simulink model "lin_mpc_qpoases_inline"  (Simulink 7.8)
settings: Solver=ode45  StartTime=0.0  StopTime=300  RelTol=1e-3
values from neighbouring files (symbols this model uses):
  x_init_lin = [0.898 ... (first row only)    [MpcSetup.m]    (also in MpcSetup_linearized.m; compressor_setup.m; setup_compressor.m; test2.m = [0.899; 1.125; 0.1512; 440.7; 0])
settings Model: Creator=CHANCOR1  LastModifiedBy=chkajon
settings DebuggingCC: FcnCallInpInsideContextMsg=Use local settings  StrictBusMsg=Warning
settings SFSimCC: SimUserSources=../call_qpoases_m/call_qpoases.c
settings SFSimCC: SimUserIncludeDirs=|
  | ../call_qpoases_m/qpoases3/src
  | ../call_qpoases_m/qpoases3/include

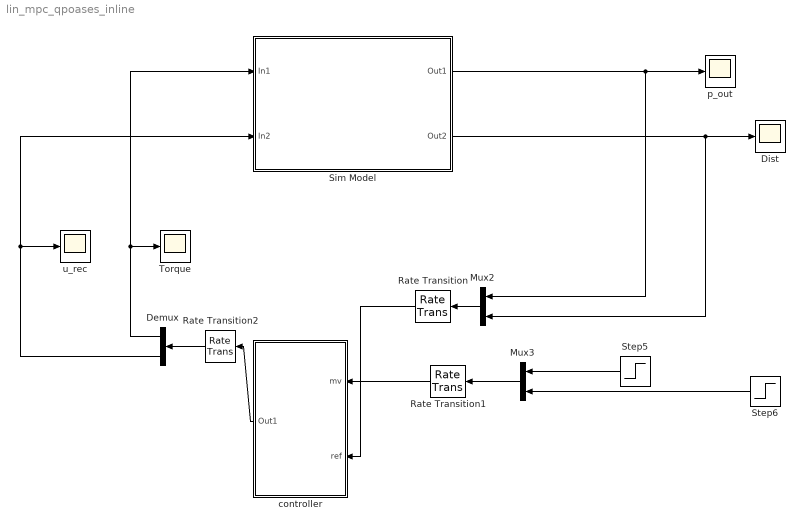
== system lin_mpc_qpoases_inline ==
  Demux : Demux  Outputs=2
  Dist : Scope
      settings: TimeRange=300  YMin=-0.3  YMax=0.1  SaveName=SD  DataFormat=Array
  Mux2 : Mux  Inputs=2
  Mux3 : Mux  Inputs=2
  Rate Transition : RateTransition  X0=[1.126; 0.046]
  Rate Transition1 : RateTransition
  Rate Transition2 : RateTransition
  Sim Model : Subsystem
  Step5 : Step  Time=30  After=0  SampleTime=0
  Step6 : Step  Time=30  After=0  SampleTime=0
  Torque : Scope
      settings: TimeRange=300  YMin=-0.125  YMax=0.125  SaveName=ScopeData17
  controller : Subsystem
  p_out : Scope
      settings: TimeRange=300  YMin=-0.05  YMax=0.225  SaveName=ScopeData3
  u_rec : Scope
      settings: TimeRange=300  YMin=-3.46945e-018  YMax=0.1
  wires:
  Step5/1 -> Mux3/1
  Step6/1 -> Mux3/2
  Demux/1 -> Torque/1, Sim Model/1(In1)
  controller/1(Out1) -> Rate Transition2/1
  Mux2/1 -> Rate Transition/1
  Mux3/1 -> Rate Transition1/1
  Rate Transition/1 -> controller/1(mv)
  Rate Transition1/1 -> controller/2(ref)
  Rate Transition2/1 -> Demux/1
  Demux/2 -> Sim Model/2(In2), u_rec/1
  Sim Model/2(Out2) -> Dist/1, Mux2/2
  Sim Model/1(Out1) -> p_out/1, Mux2/1

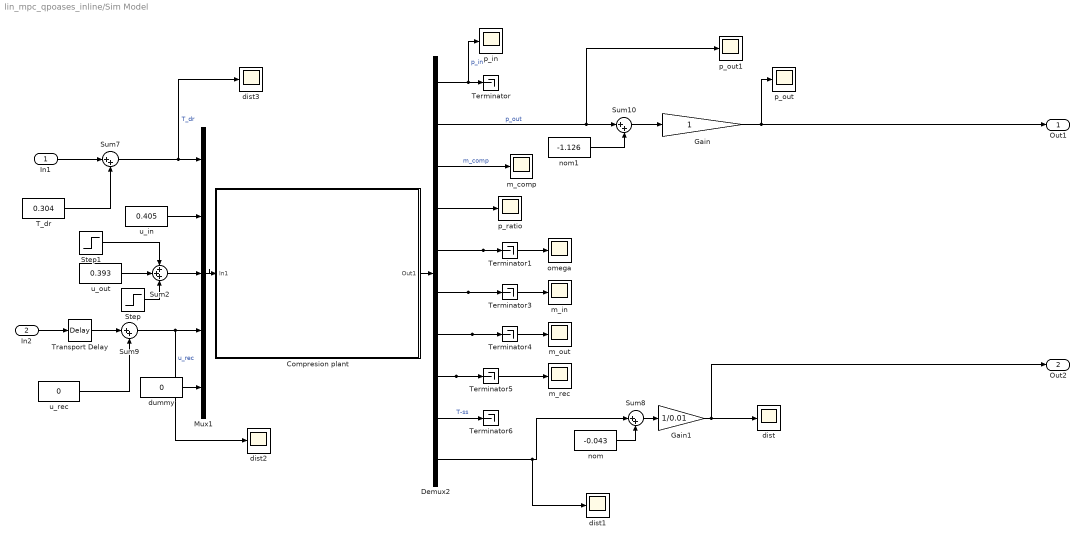
== system lin_mpc_qpoases_inline/Sim Model ==
  In1 : Inport
  In2 : Inport  Port=2
  Compresion plant : Subsystem
      mask Display: image(imread('comp_plant.jpg'))
  Demux2 : Demux  Outputs=10
  Gain : Gain
  Gain1 : Gain  Gain=1/0.01
  Mux1 : Mux  Inputs=5
  Step : Step  Time=50  After=-0.1  SampleTime=0
  Step1 : Step  Time=100  After=-0.1  SampleTime=0
  Sum{7..10} (4 alike) : Sum  Inputs=|++
  Sum2 : Sum  Inputs=+++
  T_dr : Constant  Value=0.304
  Terminator{,1,3..6} (6 alike) : Terminator
  Transport Delay : TransportDelay  DelayTime=1.0
  dist{,1..3} (4 alike) : Scope
      dist settings: YMin=-11  YMax=2  SaveName=ScopeData6
      dist1 settings: TimeRange=100  YMin=0.03  YMax=0.075  SaveName=ScopeData5
      dist2 settings: TimeRange=100  YMin=-0.25  YMax=1  SaveName=ScopeData4
      dist3 settings: TimeRange=100  YMin=-9  YMax=1  SaveName=ScopeData2
  dummy : Constant  Value=0
  m_comp : Scope
      settings: TimeRange=100  YMin=0.5  YMax=0.825  SaveName=m_comp  DataFormat=Array
  m_in : Scope
      settings: TimeRange=100  YMin=100.8  YMax=100.975  SaveName=ScopeData11
  m_out : Scope
      settings: TimeRange=100  YMin=100.8  YMax=100.975  SaveName=ScopeData12
  m_rec : Scope
      settings: TimeRange=100  YMin=100.8  YMax=100.975  SaveName=ScopeData13
  nom : Constant  Value=-0.043
  nom1 : Constant  Value=-1.126
  omega : Scope
      settings: TimeRange=100  YMin=200  YMax=700  SaveName=ScopeData10
  p_in : Scope
      settings: TimeRange=100  YMin=0.895197  YMax=0.895225  SaveName=ScopeData9
  p_out : Scope
      settings: TimeRange=100  YMin=-2.5  YMax=40  SaveName=ScopeData7
  p_out1 : Scope
      settings: TimeRange=100  YMin=100.8  YMax=100.975  SaveName=ScopeData8
  p_ratio : Scope
      settings: TimeRange=100  YMin=0.5  YMax=0.825  SaveName=p_ratio  DataFormat=Array
  u_in : Constant  Value=0.405
  u_out : Constant  Value=0.393
  u_rec : Constant  Value=0
  Out1 : Outport
  Out2 : Outport  Port=2
  wires:
  Demux2/9 -> Terminator6/1  "T-ss"
  Sum2/1 -> Mux1/3
  Step/1 -> Sum2/3
  Transport Delay/1 -> Sum9/1
  dummy/1 -> Mux1/5
  Demux2/10 -> dist1/1, Sum8/1
  Gain1/1 -> dist/1, Out2/1
  In1/1 -> Sum7/1
  u_rec/1 -> Sum9/2
  T_dr/1 -> Sum7/2
  Gain/1 -> p_out/1, Out1/1
  nom1/1 -> Sum10/2
  Sum10/1 -> Gain/1
  Demux2/4 -> p_ratio/1
  Demux2/5 -> omega/1, Terminator1/1
  Demux2/1 -> p_in/1, Terminator/1  "p_in"
  Demux2/2 -> p_out1/1, Sum10/1  "p_out"
  Sum8/1 -> Gain1/1
  nom/1 -> Sum8/2
  Sum9/1 -> dist2/1, Mux1/4  "u_rec"
  Sum7/1 -> Mux1/1, dist3/1  "T_dr"
  In2/1 -> Transport Delay/1
  u_out/1 -> Sum2/2
  Demux2/7 -> m_out/1, Terminator4/1
  Demux2/8 -> m_rec/1, Terminator5/1
  Demux2/6 -> m_in/1, Terminator3/1
  u_in/1 -> Mux1/2
  Demux2/3 -> m_comp/1  "m_comp"
  Mux1/1 -> Compresion plant/1(In1)
  Compresion plant/1(Out1) -> Demux2/1
  Step1/1 -> Sum2/1

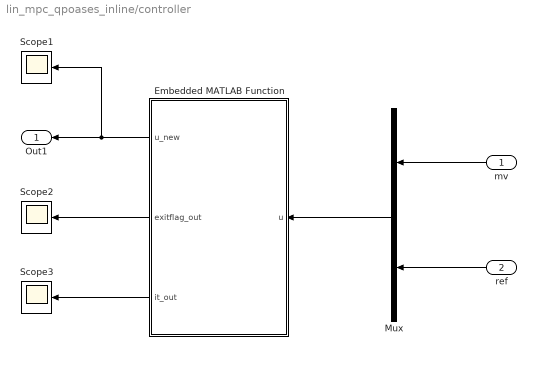
== system lin_mpc_qpoases_inline/controller ==
  mv : Inport
  ref : Inport  Port=2
  Embedded MATLAB Function : MATLAB Function  TreatAsAtomicUnit=on  SystemSampleTime=0.05
  Mux : Mux  Inputs=2
  Scope1 : Scope
      settings: YMin=0  YMax=0.6
  Scope2 : Scope
      settings: YMin=-1  YMax=1  SaveName=ScopeData15
  Scope3 : Scope
      settings: YMin=10  YMax=47.5  SaveName=ScopeData16
  Out1 : Outport
  wires:
  mv/1 -> Mux/1
  Mux/1 -> Embedded MATLAB Function/1(u)
  ref/1 -> Mux/2
  Embedded MATLAB Function/1(u_new) -> Out1/1, Scope1/1
  Embedded MATLAB Function/3(it_out) -> Scope3/1
  Embedded MATLAB Function/2(exitflag_out) -> Scope2/1

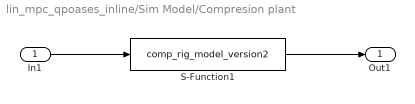
== system lin_mpc_qpoases_inline/Sim Model/Compresion plant ==
  In1 : Inport
  S-Function1 : S-Function  FunctionName=comp_rig_model_version2  Parameters=[], x_init_lin  EnableBusSupport=off
  Out1 : Outport
  wires:
  In1/1 -> S-Function1/1
  S-Function1/1 -> Out1/1

== matlab function controller/Embedded MATLAB Function ==
  data: u input double; u_new output double; exitflag_out output double; it_out output double
function [u_new,exitflag_out,it_out]  = fcn(u)
%#eml
persistent C_new M LB UB Ga Gb Gc H Ain b A B upast xinit
eml.extrinsic('disp');
eml.extrinsic('toc');
eml.extrinsic('tic');
eml.extrinsic('num2str');
eml.extrinsic('keyboard');

p=200;
m=8;
usize = 2;
ysize = 2;
% p = 100;
% m = 10;

if isempty(M)
    tic
    option = 1;
    [H,C_new,M,UB,LB,b,Ain,Ga,Gb,Gc,xinit,upast] = get_matrices(option);
%     xinit(1:4,1) = [0.8980 1.1260 0.1500 439.5000]';
    [A,B] = get_matAB(option);
    
    time = toc;
    disp(['Preparation time: ' num2str(time)]);
end

% get the measurements for outputs and the output reference
y=u(1:2);
yref=u(3:4);

% estimate the state information
xinit  = xinit + M*(y(:) - C_new*xinit);

% upper/lower bounds wrt past input
% Upast = repmat(upast,m,1);
Upast = zeros(usize*m,1);
for i=1:m
    Upast(1+(i-1)*usize:i*usize,1) = upast;
end

LBa = LB - Upast;
UBa = UB - Upast;

% Reference output vector
% Yref = repmat(yref,p,1);
Yref = zeros(ysize*p,1);
for i=1:p
    Yref(1+(i-1)*ysize:i*ysize,1) = yref;
end

% define f vector for qp
f = xinit' * Gb + Upast'*Gc - Yref' * Ga;

% solve qp
lbA = -inf*ones(size(Ain,1));
[usol,cost,exitflag,it,lambda] = call_qpoases_m(H,f,Ain,LBa,UBa,lbA,b);
exitflag_out = exitflag(1,1);
it_out = it(1,1);
next = usol(1:usize,1);

% update state estimate
xinit= A*xinit + B*(upast+next);

% update next control move
upast = upast + next;


u_new=upast;

% tic

% H_star = H;
% % H_star = (H+H')/2;
% Ain_star = Ain;
% b_star = b;
% 
% y=u(1:2);
% yref=u(3:4);
% 
% 
% %%%%%%%%%%%%%%%%%%%%%%%%%%%%%%%%%%%%%%%%%%%%%%%%%%%%%%%%%%
% 
% 
% % estimate the state information
% 
% 
% xinit  = xinit + M*(y - C_new*xinit);
% 
% %%%%%%%%%%%%%%%%%%%%%%%%%%%%%%%%%%%%%%%%%%%%%%%%%%%%%%%%%%
% 
% % upper and lower bounds wrt past input
% Upast = zeros(m*2,1);
% 
% for i=1:m
%     Upast(1+(i-1)*2:i*2,1)=upast;
% end
% 
% LBa=LB-Upast;
% UBa=UB-Upast;
% 
% 
% 
% %%%%%%%%%%%%%%%%%%%%%%%%%%%%%%%%%%%%%%%%%%%%%%%%%%%%%%%%%%
% 
% % generate the output reference vector
% 
% R = zeros(p*2,1);
% 
% for i=1:p
%     R(1+(i-1)*2:i*2,1)=yref;
% end
% 
% % generate the gradient vector
% 
% f = xinit'*Gb+Upast'*Gc-R'*Ga;
% 
% % xinit1 = xinit;
% % upast1 = upast;
% 
% lbA = [-inf(size(Ain_star,1),1)];
% ubA = [b_star];
% [usol,cost,exitflag,it,lambda] = call_qpoases_m(H_star,f,Ain_star,LBa,UBa,lbA,ubA);
% exitflag_out = exitflag(1,1);
% it_out = it(1,1);
% dunext=usol(1:2,1);
% 
% xinit= A*xinit + B*(dunext+upast);
% 
% u_new=dunext+upast;
% 
% upast = u_new;

% time2 = toc;
% disp(['Normal Execution Time: ' num2str(time2)]);
%%%%%%%%%%%%%%%%%%%%%%%%%%%%%%%%%%%%%%%%%%%%%%%%%%%%%%%%%%


% solve the QP

% usol=quadprog(H_qp,f,Ain,b,[],[],LBa,UBa);
% 
% 
% %%%%%%%%%%%%%%%%%%%%%%%%%%%%%%%%%%%%%%%%%%%%%%%%%%%%%%%%%%
% 
% 
% % extract the control moves for next time step
% 
% 
% dunext=usol(1:2,1);
% 
% 
% %%%%%%%%%%%%%%%%%%%%%%%%%%%%%%%%%%%%%%%%%%%%%%%%%%%%%%%%%%
% 
% 
% % initial conditions are updated
% 
% 
% xinit= A*xinit + B*(dunext+upast);
% 
% 
% %%%%%%%%%%%%%%%%%%%%%%%%%%%%%%%%%%%%%%%%%%%%%%%%%%%%%%%%%%
% 
% % control moves are sent to the plant
% 
% upast=dunext+upast;
% 
% sys=upast;
